simulink model "trackCirc"  (R2020a)
settings: Solver=VariableStepAuto  StartTime=0.0  StopTime=180  RelTol=1e-8
undefined symbols (not defined in the file or in its folder): A_latFor, B_latFor, C_latFor, den_long, IC, K, L, num_long, sensor_gain
libraries: simulink x1
settings Model: Creator=Tomo  LastModifiedBy=Tomo

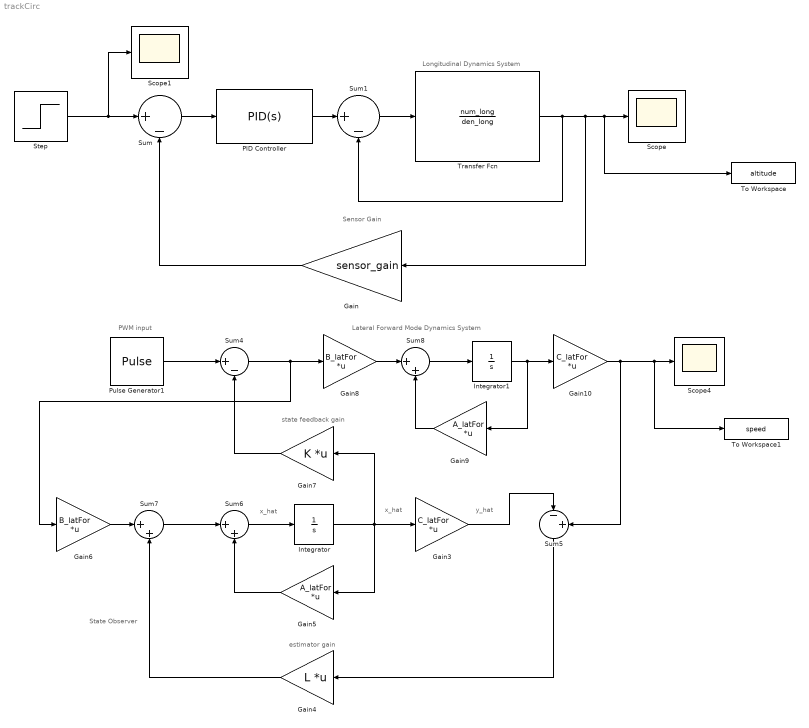
== system trackCirc ==
  note: Sensor Gain
  note: Longitudinal Dynamics System
  note: estimator gain
  note: y_hat
  note: x_hat
  note: Lateral Forward Mode Dynamics System
  note: state feedback gain
  note: x_hat
  note: State Observer
  note: PWM input
  Gain : Gain  Gain=sensor_gain
  Gain10 : Gain  Gain=C_latFor  Multiplication=Matrix(K*u)
  Gain3 : Gain  Gain=C_latFor  Multiplication=Matrix(K*u)
  Gain4 : Gain  Gain=L  Multiplication=Matrix(K*u)
  Gain5 : Gain  Gain=A_latFor  Multiplication=Matrix(K*u)
  Gain6 : Gain  Gain=B_latFor  Multiplication=Matrix(K*u)
  Gain7 : Gain  Gain=K  Multiplication=Matrix(K*u)
  Gain8 : Gain  Gain=B_latFor  Multiplication=Matrix(K*u)
  Gain9 : Gain  Gain=A_latFor  Multiplication=Matrix(K*u)
  Integrator : Integrator  InitialCondition=IC
  Integrator1 : Integrator  InitialCondition=IC
  PID Controller : simulink/Continuous/PID Controller  Controller=PID  Form=Parallel  TimeDomain=Continuous-time  UseExternalTs=off  SampleTime=-1  IntegratorMethod=Forward Euler  FilterMethod=Forward Euler  ControllerParametersSource=internal  P=-0.307379439514045  I=1.76787636529414  D=0.784330846762679  UseFilter=on  N=3.38233444179698  TunerSelectOption=Transfer Function Based (PID Tuner App)  InitialConditionSource=internal  InitialConditionForIntegrator=0  InitialConditionForFilter=0  DifferentiatorICPrevScaledInput=0  ExternalReset=none  TrackingMode=off  Kt=1  LimitOutput=off  UpperSaturationLimit=inf  LowerSaturationLimit=-inf  LinearizeAsGain=on  AntiWindupMode=none  Kb=1  POutMin=[]  POutMax=[]  IOutMin=[]  IOutMax=[]  DOutMin=[]  DOutMax=[]  NOutMin=[]  NOutMax=[]  SumOutMin=[]  SumOutMax=[]  SaturationOutMin=[]  SaturationOutMax=[]  PParamMin=[]  PParamMax=[]  IParamMin=[]  IParamMax=[]  DParamMin=[]  DParamMax=[]  NParamMin=[]  NParamMax=[]  KbParamMin=[]  KbParamMax=[]  KtParamMin=[]  KtParamMax=[]  KbOutMin=[]  KbOutMax=[]  KtOutMin=[]  KtOutMax=[]  IntegratorOutMin=[]  IntegratorOutMax=[]  FilterOutMin=[]  FilterOutMax=[]  SumI1OutMin=[]  SumI1OutMax=[]  SumI2OutMin=[]  SumI2OutMax=[]  SumI3OutMin=[]  SumI3OutMax=[]  SumI4OutMin=[]  SumI4OutMax=[]  SumDOutMin=[]  SumDOutMax=[]  DifferentiatorOutMin=[]  DifferentiatorOutMax=[]  FilterDiffOutCoefMin=[]  FilterDiffOutCoefMax=[]  ReciprocalOutMin=[]  ReciprocalOutMax=[]  SumDenOutMin=[]  SumDenOutMax=[]  SumNumOutMin=[]  SumNumOutMax=[]  DivideOutMin=[]  DivideOutMax=[]  UdiffTsProdOutMin=[]  UdiffTsProdOutMax=[]  NTsProdOutMin=[]  NTsProdOutMax=[]  UintegralTsProdOutMin=[]  UintegralTsProdOutMax=[]  UngainTsProdOutMin=[]  UngainTsProdOutMax=[]  IntegratorContinuousStateAttributes=''  IntegratorStateMustResolveToSignalObject=off  IntegratorRTWStateStorageClass=Auto  FilterContinuousStateAttributes=''  FilterStateMustResolveToSignalObject=off  FilterRTWStateStorageClass=Auto  ParallelPVariant=InternalParameters  IdealPVariant=Disabled  IVariant=InternalParameters  DVariant=InternalParameters  IntegratorVariant=Continuous  SatVariant=Disabled  AWVariant=Passthrough  PCopyVariant=Disabled  TRVariant=Disabled  FdbkBlocksVariant=Forward  IdealPFdbkVariant=Disabled  SatFdbkVariant=Disabled  DerivativeFilterVariant=ContFilter  NVariant=InternalParameters  NCopyVariant=Disabled  FilterICVariant=InternalICsFilter  IntegratorICVariant=InternalICs  ExternalResetVariant=Disabled  TRSumVariant=Passthrough  SumFdbkVariant=Disabled  SumVariant=Sum_PID  TsampFilterVariant=InternalTs  TsampNgainVariant=Passthrough  TsampIntegralVariant=Passthrough
  Pulse Generator1 : DiscretePulseGenerator  PulseType=Time based  Amplitude=100  Period=1/50  PulseWidth=99.9999
  Scope : Scope
  Scope1 : Scope
  Scope4 : Scope
  Step : Step  After=1000  SampleTime=0
  Sum : Sum  Inputs=|+-
  Sum1 : Sum  Inputs=|+-
  Sum4 : Sum  Inputs=|+-
  Sum5 : Sum  Inputs=|-+
  Sum6 : Sum  Inputs=|++
  Sum7 : Sum  Inputs=|++
  Sum8 : Sum  Inputs=|++
  To Workspace : ToWorkspace  VariableName=altitude  SaveFormat=Structure With Time  SampleTime=-1
  To Workspace1 : ToWorkspace  VariableName=speed  SaveFormat=Structure With Time  SampleTime=-1
  Transfer Fcn : TransferFcn  Numerator=num_long  Denominator=den_long
  wires:
  PID Controller/1 -> Sum1/1
  Sum/1 -> PID Controller/1
  Gain/1 -> Sum/2
  Sum1/1 -> Transfer Fcn/1
  Transfer Fcn/1 -> Sum1/2, Gain/1, To Workspace/1, Scope/1
  Sum6/1 -> Integrator/1
  Gain5/1 -> Sum6/2
  Sum5/1 -> Gain4/1
  Gain4/1 -> Sum7/2
  Sum4/1 -> Gain8/1, Gain6/1
  Gain10/1 -> Sum5/2, To Workspace1/1, Scope4/1
  Integrator/1 -> Gain5/1, Gain7/1, Gain3/1
  Gain9/1 -> Sum8/2
  Gain6/1 -> Sum7/1
  Sum7/1 -> Sum6/1
  Gain8/1 -> Sum8/1
  Gain7/1 -> Sum4/2
  Gain3/1 -> Sum5/1
  Pulse Generator1/1 -> Sum4/1
  Integrator1/1 -> Gain9/1, Gain10/1
  Sum8/1 -> Integrator1/1
  Step/1 -> Scope1/1, Sum/1
